simulink library "INT_FanSpd_DD"  (R2016b)
settings: Solver=VariableStepAuto  StartTime=0.0  StopTime=10.0  RelTol=1e-3
settings Model: Creator=xinchangran  LastModifiedBy=xinchangran

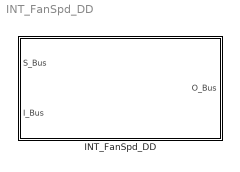
== system INT_FanSpd_DD ==
  INT_FanSpd_DD : Subsystem

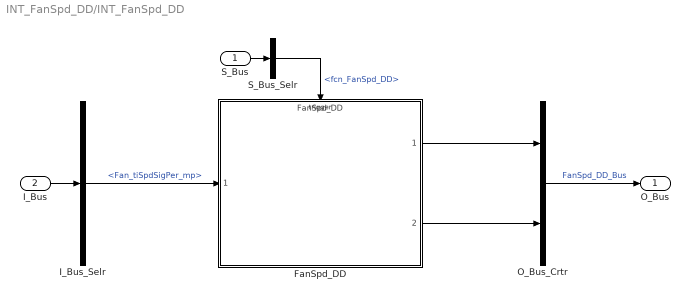
== system INT_FanSpd_DD/INT_FanSpd_DD ==
  S_Bus : Inport
  I_Bus : Inport  Port=2
  FanSpd_DD : ModelReference  ModelNameDialog=FanSpd_DD  SimulationMode=Normal  ModelReferenceVersion=1.51  TriggerPortName=function  TriggerPortTriggerType=function-call  TriggerPortStatesWhenEnabling=held
  I_Bus_Selr : BusSelector  OutputSignals=Fan_tiSpdSigPer_mp
  O_Bus_Crtr : BusCreator  Inputs=2
  S_Bus_Selr : BusSelector  OutputSignals=fcn_FanSpd_DD
  O_Bus : Outport
  wires:
  S_Bus_Selr/1 -> FanSpd_DD/Trigger  "<fcn_FanSpd_DD>"
  S_Bus/1 -> S_Bus_Selr/1
  I_Bus/1 -> I_Bus_Selr/1
  I_Bus_Selr/1 -> FanSpd_DD/1  "<Fan_tiSpdSigPer_mp>"
  O_Bus_Crtr/1 -> O_Bus/1  "FanSpd_DD_Bus"
  FanSpd_DD/1 -> O_Bus_Crtr/1
  FanSpd_DD/2 -> O_Bus_Crtr/2
